simulink model "QuadTank_MPC"  (R2019b)
settings: Solver=ode45  StartTime=0.0  StopTime=1500  RelTol=1e-3  EnableMultiTasking=on
values from neighbouring files (symbols this model uses):
  a1 = Ao1    (= 0.17813934812)    [Process_data.m]    (also in Process_setup.m; QuadTankDriver.m = Ao1; Simulate_QuadTank_MPC_LECO.m)
  A1 = At1    (= 15.5179165474)    [Process_data.m]    (also in Process_setup.m; QuadTankDriver.m = At1; Simulate_QuadTank_MPC_LECO.m)
  a2 = Ao2    (= 0.17813934812)    [Process_data.m]    (also in Process_setup.m; QuadTankDriver.m = Ao2; Simulate_QuadTank_MPC_LECO.m)
  A2 = At2    (= 15.5179165474)    [Process_data.m]    (also in Process_setup.m; QuadTankDriver.m = At2; Simulate_QuadTank_MPC_LECO.m)
  a3 = Ao3    (= 0.17813934812)    [Process_data.m]    (also in Process_setup.m; QuadTankDriver.m = Ao3; Simulate_QuadTank_MPC_LECO.m)
  A3 = At3    (= 15.5179165474)    [Process_data.m]    (also in Process_setup.m; QuadTankDriver.m = At3; Simulate_QuadTank_MPC_LECO.m)
  a4 = Ao4    (= 0.17813934812)    [Process_data.m]    (also in Process_setup.m; QuadTankDriver.m = Ao4; Simulate_QuadTank_MPC_LECO.m)
  A4 = At4    (= 15.5179165474)    [Process_data.m]    (also in Process_setup.m; QuadTankDriver.m = At4; Simulate_QuadTank_MPC_LECO.m)
  g = 981    [Process_data.m]    (also in Process_setup.m; Simulate_QuadTank_MPC_LECO.m)
  g1_nmp = gamma1    (= 0.64)    [Process_data.m]    (also in Process_setup.m; QuadTankDriver.m = gamma1; Simulate_QuadTank_MPC_LECO.m)
  g2_nmp = gamma2    (= 0.64)    [Process_data.m]    (also in Process_setup.m; QuadTankDriver.m = gamma2; Simulate_QuadTank_MPC_LECO.m)
  h10_nmp = L10    [QuadTankDriver.m]    (also in Simulate_QuadTank_MPC_LECO.m = 10)
  h20_nmp = L20    [QuadTankDriver.m]    (also in Simulate_QuadTank_MPC_LECO.m = 14)
  h30_nmp = L30    [QuadTankDriver.m]    (also in Simulate_QuadTank_MPC_LECO.m = ((1-gamma2)*Kp*v20_nmp/Ao3)^2/(2*g))
  h40_nmp = L40    [QuadTankDriver.m]    (also in Simulate_QuadTank_MPC_LECO.m = ((1-gamma1)*Kp*v10_nmp/Ao4)^2/(2*g))
  k1_nmp = 3.3    [Process_data.m]    (also in Process_setup.m; QuadTankDriver.m = Kp; Simulate_QuadTank_MPC_LECO.m)
  k2_nmp = 3.3    [Process_data.m]    (also in Process_setup.m; QuadTankDriver.m = Kp; Simulate_QuadTank_MPC_LECO.m)
  kc = 4.15/25    (= 0.166)    [Process_data.m]    (also in Process_setup.m; Simulate_QuadTank_MPC_LECO.m)
  md = MPCInit(Ad,Bd,Cyd,Czd,Dzd,Ccd,Dcd,Hp,Hw,zblk,Hu,ublk,  	    du_max,du_min,u_max,u_min,z_max,  	    z_min,Q,R,W,V,h,4,'qp_as')    [Simulate_QuadTank_MPC_LECO.m]
  v10_nmp = Vp10    [QuadTankDriver.m]    (also in Simulate_QuadTank_MPC_LECO.m = Ao1*sqrt(2*g*h10_nmp)/(gamma1*Kp)-(1-gamma2)*v20_nmp/gamma1)
  v20_nmp = Vp20    [QuadTankDriver.m]    (also in Simulate_QuadTank_MPC_LECO.m = Ao1*(1-gamma1)*sqrt(2*g*h10_nmp)/(((1-gamma1)*(1-gamma2)-gam)
undefined symbols (not defined in the file or in its folder): QuadTank
settings Model: ExtModeAutoUpdateStatusClock=off  Creator=jakesson  LastModifiedBy=adegbega
settings DataIOCC: LimitDataPoints=on  SaveFormat=Array  SignalLoggingSaveFormat=ModelDataLogs  ReturnWorkspaceOutputs=off  SignalLoggingName=sigsOut
settings OptimizationCC: BooleanDataType=off  InitFltsAndDblsToZero=on  LifeSpan=inf
settings DebuggingCC: SaveWithParameterizedLinksMsg=none  UnderspecifiedInitializationDetection=Classic  MergeDetectMultiDrivingBlocksExec=none  SignalResolutionControl=TryResolveAllWithWarning  MultiTaskDSMMsg=warning  MultiTaskCondExecSysMsg=none  FcnCallInpInsideContextMsg=warning  SFUnexpectedBacktrackingDiag=warning  SFNoUnconditionalDefaultTransitionDiag=warning  SFExecutionAtInitializationDiag=none  ArithmeticOperatorsInVariantConditions=warning
settings HardwareCC: ProdBitPerPointer=32  ProdBitPerSizeT=32  ProdBitPerPtrDiffT=32  ProdLargestAtomicFloat=None  ProdIntDivRoundTo=Undefined  ProdEndianess=Unspecified  ProdWordSize=32  ProdHWDeviceType=32-bit Generic  TargetUnknown=on
settings ModelReferenceCC: PropagateSignalLabelsOutOfModel=off
settings CodeAppCC: StateflowObjectComments=on
settings GRTTargetCC: TargetFcnLib=ansi_tfl_tmw.mat  TargetLangStandard=C89/C90 (ANSI)  CombineOutputUpdateFcns=off  GRTInterface=on
settings ConfigComp: CovMetricSettings=dw  CovHtmlReporting=on  CovSaveCumulativeToWorkspaceVar=on  CovSaveSingleToWorkspaceVar=on

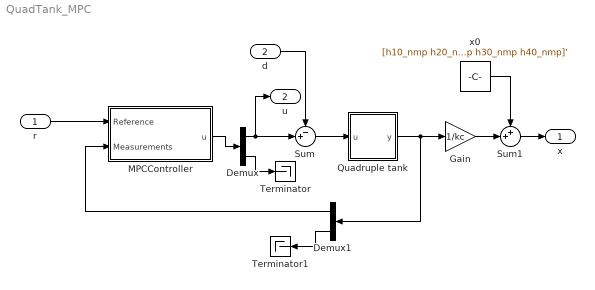
== system QuadTank_MPC ==
  r : Inport
  d : Inport  Port=2  PortDimensions=2
  Demux : Demux  Outputs=[md.m md.ne]
  Demux1 : Demux  Outputs=[2 2]
  Gain : Gain  Gain=1/kc  SaturateOnIntegerOverflow=on  OutDataTypeStr=Inherit: Same as input  ParamDataTypeStr=Inherit: Same as input
  MPCController : Subsystem  mask{md=md}
      mask prompts: md "MPCData"
  Quadruple tank : Subsystem
  Sum : Sum  Inputs=-+|  SaturateOnIntegerOverflow=on  InputSameDT=on  OutDataTypeStr=Inherit: Same as first input
  Sum1 : Sum  Inputs=++|  SaturateOnIntegerOverflow=on  InputSameDT=on  OutDataTypeStr=Inherit: Same as first input
  Terminator : Terminator
  Terminator1 : Terminator
  x0 : Constant  Value=[h10_nmp h20_nmp h30_nmp h40_nmp]'
  x : Outport
  u : Outport  Port=2
  wires:
  MPCController/1(u) -> Demux/1
  Sum/1 -> Quadruple tank/1(u)
  d/1 -> Sum/1
  Demux/1 -> Sum/2, u/1
  r/1 -> MPCController/1(Reference)
  Quadruple tank/1(y) -> Gain/1, Demux1/1
  Demux/2 -> Terminator/1
  Demux1/2 -> Terminator1/1
  Sum1/1 -> x/1
  Gain/1 -> Sum1/2
  x0/1 -> Sum1/1
  Demux1/1 -> MPCController/2(Measurements)

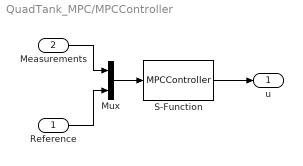
== system QuadTank_MPC/MPCController ==
  Reference : Inport
  Measurements : Inport  Port=2
  Mux : Mux  Inputs=2
  S-Function : S-Function  FunctionName=MPCController  Parameters=md  SFunctionDeploymentMode=off  EnableBusSupport=off
  u : Outport
  wires:
  Mux/1 -> S-Function/1
  Measurements/1 -> Mux/1
  Reference/1 -> Mux/2
  S-Function/1 -> u/1

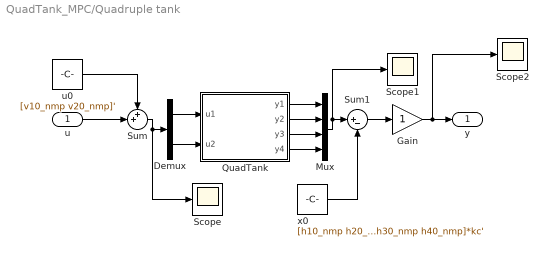
== system QuadTank_MPC/Quadruple tank ==
  u : Inport
  Demux : Demux  Outputs=2
  Gain : Gain  SaturateOnIntegerOverflow=on  OutDataTypeStr=Inherit: Same as input  ParamDataTypeStr=Inherit: Same as input
  Mux : Mux
  QuadTank : Subsystem  AncestorBlock=QuadTank/QuadTank  mask{h0=[0 0 0 0]', g1=g1_nmp, g2=g2_nmp, k1=k1_nmp, k2=k2_nmp}
      mask prompts: h0 "Initial levels"; g1 "Valve 1"; g2 "Valve 2"; k1 "Pump coefficient 1"; k2 "Pump coefficient 2"
  Scope : Scope
  Scope1 : Scope
  Scope2 : Scope
  Sum : Sum  Inputs=++|  SaturateOnIntegerOverflow=on  InputSameDT=on  OutDataTypeStr=Inherit: Same as first input
  Sum1 : Sum  Inputs=|+-  SaturateOnIntegerOverflow=on  InputSameDT=on  OutDataTypeStr=Inherit: Same as first input
  u0 : Constant  Value=[v10_nmp v20_nmp]'
  x0 : Constant  Value=[h10_nmp h20_nmp h30_nmp h40_nmp]*kc'
  y : Outport
  wires:
  Mux/1 -> Scope1/1, Sum1/1
  Sum1/1 -> Gain/1
  x0/1 -> Sum1/2
  u/1 -> Sum/2
  u0/1 -> Sum/1
  Sum/1 -> Scope/1, Demux/1
  QuadTank/2(y2) -> Mux/2
  QuadTank/1(y1) -> Mux/1
  Demux/2 -> QuadTank/2(u2)
  Demux/1 -> QuadTank/1(u1)
  Gain/1 -> Scope2/1, y/1
  QuadTank/3(y3) -> Mux/3
  QuadTank/4(y4) -> Mux/4

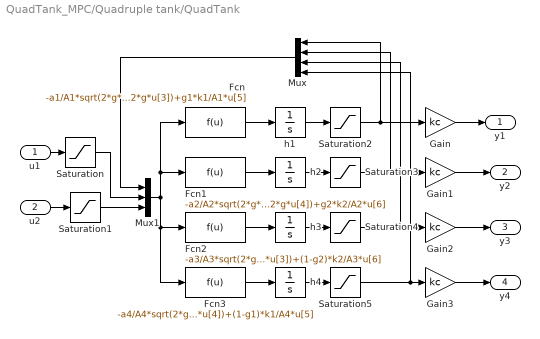
== system QuadTank_MPC/Quadruple tank/QuadTank ==
  u1 : Inport
  u2 : Inport  Port=2
  Fcn : Fcn  Expr=-a1/A1*sqrt(2*g*u[1])+a3/A1*sqrt(2*g*u[3])+g1*k1/A1*u[5]
  Fcn1 : Fcn  Expr=-a2/A2*sqrt(2*g*u[2])+a4/A2*sqrt(2*g*u[4])+g2*k2/A2*u[6]
  Fcn2 : Fcn  Expr=-a3/A3*sqrt(2*g*u[3])+(1-g2)*k2/A3*u[6]
  Fcn3 : Fcn  Expr=-a4/A4*sqrt(2*g*u[4])+(1-g1)*k1/A4*u[5]
  Gain{,1..3} (4 alike) : Gain  Gain=kc  SaturateOnIntegerOverflow=on  OutDataTypeStr=Inherit: Same as input  ParamDataTypeStr=Inherit: Same as input
  Mux : Mux
  Mux1 : Mux  Inputs=3
  Saturation : Saturate  UpperLimit=10  LowerLimit=0
  Saturation1 : Saturate  UpperLimit=10  LowerLimit=0
  Saturation{2..5} (4 alike) : Saturate  UpperLimit=50  LowerLimit=0
  h1 : Integrator  InitialCondition=h0(1)
  h2 : Integrator  InitialCondition=h0(2)
  h3 : Integrator  InitialCondition=h0(3)
  h4 : Integrator  InitialCondition=h0(4)
  y1 : Outport
  y2 : Outport  Port=2
  y3 : Outport  Port=3
  y4 : Outport  Port=4
  wires:
  Mux1/1 -> Fcn3/1, Fcn2/1, Fcn1/1, Fcn/1
  Fcn3/1 -> h4/1
  Fcn2/1 -> h3/1
  Fcn1/1 -> h2/1
  Fcn/1 -> h1/1
  u2/1 -> Saturation1/1
  u1/1 -> Saturation/1
  Mux/1 -> Mux1/1
  h2/1 -> Saturation3/1
  h1/1 -> Saturation2/1
  h3/1 -> Saturation4/1
  h4/1 -> Saturation5/1
  Gain3/1 -> y4/1
  Gain2/1 -> y3/1
  Gain1/1 -> y2/1
  Gain/1 -> y1/1
  Saturation/1 -> Mux1/2
  Saturation1/1 -> Mux1/3
  Saturation2/1 -> Mux/1, Gain/1
  Saturation3/1 -> Mux/2, Gain1/1
  Saturation4/1 -> Mux/3, Gain2/1
  Saturation5/1 -> Mux/4, Gain3/1
